simulink model "flightControlSystem"  (R2024a)
settings: Solver=ode3  StartTime=0  StopTime=1000  FixedStep=Ts  RelTol=1e-3  EnableMultiTasking=on
undefined symbols (not defined in the file): codertarget, Controller, DiscIntNeverNeededParam, Discrete, Estimator, g, gray, init, Sensors, Time, Ts, var_acc_angle_N, var_bias_gyr_N, var_gyro_p_N, Vehicle
libraries: simulink x37, slpidlib x4, ctrlSharedLib x4, sharedtransform x3, parrotlib x1
(part 3 of 3)

== matlab function flightControlSystem/Image Processing System/MATLAB Function1 ==
  data: R input; BW output; G input; B input
function BW  = createMask(R,G,B)

    % Define thresholds for channel 1 based on histogram settings
    channel1Min = 135.000;
    channel1Max = 255.000;
    
    % Define thresholds for channel 2 based on histogram settings
    channel2Min = 0.000;
    channel2Max = 112.000;
    
    % Define thresholds for channel 3 based on histogram settings
    channel3Min = 0.000;
    channel3Max = 255.000;
       
    % NO MARKERS DETECTED
    % 
    % channel1Min = 240.000;
    % channel1Max = 255.000;
    % channel2Min = 0.000;
    % channel2Max = 254.000;
    % channel3Min = 0.000;
    % channel3Max = 254.000;
    
    % % MARKERS ALSO DETECTED
    % 
    % channel1Min = 230.000;
    % channel1Max = 255.000;
    % channel2Min = 0.000;
    % channel2Max = 255.000;
    % channel3Min = 0.000;
    % channel3Max = 255.000;

    % Create mask based on chosen histogram thresholds
    sliderBW = (R >= channel1Min ) & (R <= channel1Max) & ...
        (G >= channel2Min ) & (G <= channel2Max) & ...
        (B >= channel3Min ) & (B <= channel3Max);
    BW = sliderBW;
    
    % RGB = cat(3,R,G,B);
    % maskedRGBImage = RGB;
    % 
    % % Set background pixels where BW is false to zero.
    % maskedRGBImage(repmat(~BW,[1 1 3])) = 0;

end

== matlab function flightControlSystem/Image Processing System/PROCESSED MASK ==
  data: R input; BW output; G input; B input
function BW  = createMask(R,G,B)
    R = imgaussfilt(R, 2);  % 2 is the standard deviation of the Gaussian filter
    G = imgaussfilt(G, 2);
    B = imgaussfilt(B, 2);

    R = imadjust(R);
    G = imadjust(G);
    B = imadjust(B);

    % Define thresholds for each channel based on the histogram settings
    channel1Min = 135.000;
    channel1Max = 255.000;
    channel2Min = 0.000;
    channel2Max = 112.000;
    channel3Min = 0.000;
    channel3Max = 255.000;
       
    % NO MARKERS DETECTED
    % 
    % channel1Min = 240.000;
    % channel1Max = 255.000;
    % channel2Min = 0.000;
    % channel2Max = 254.000;
    % channel3Min = 0.000;
    % channel3Max = 254.000;
    
    % % MARKERS ALSO DETECTED
    % 
    % channel1Min = 230.000;
    % channel1Max = 255.000;
    % channel2Min = 0.000;
    % channel2Max = 255.000;
    % channel3Min = 0.000;
    % channel3Max = 255.000;

    % Create mask based on chosen histogram thresholds
    sliderBW = (R >= channel1Min ) & (R <= channel1Max) & ...
        (G >= channel2Min ) & (G <= channel2Max) & ...
        (B >= channel3Min ) & (B <= channel3Max);

    BW = sliderBW;
    
    BW = bwareaopen(BW, 50);  % Remove small objects with area less than 50 pixels

    BW = imfill(BW, 'holes');

    se = strel('disk', 3);  % Structural element for morphological operations
    BW = imclose(BW, se);   % Close gaps in the mask
    BW = imopen(BW, se);    % Remove small objects

end
